simulink model "DFIG_and_BESS_Voltae_Control"  (R2017b)
settings: Solver=ode45  StartTime=0.0  StopTime=6  RelTol=1e-3  EnableMultiTasking=on
undefined symbols (not defined in the file): beta, Cbus, cp_opt_abs, D, D1, D11, Delta, DiscIntNeverNeededParam, f, Fs, fsw, Ion, J, ki_id, ki_idg, ki_iq, ki_iqg, ki_v, kp_id, kp_idg, kp_iq, kp_iqg, kp_v, Kpg, Kqg, lambda_opt, Lg, Lithium, Lm, Lr, Ls, Lsi, N, p, Ps, Radio, Rg, ro, Rr, Rs, sigbuilder_block, sigma, Ts, Vbus_ref, Vdc_bat_ref, Vs
libraries: powerlib x62, powerlib_meascontrol x30, electricdrivelib x1, sps_avr x1
(part 1 of 2)
settings Model: SimulationMode=accelerator  Creator=admin  LastModifiedBy=admin
settings DataIOCC: LimitDataPoints=on  SaveFormat=Array
settings OptimizationCC: EfficientMapNaN2IntZero=off  LifeSpan=inf
settings DebuggingCC: UnderspecifiedInitializationDetection=Classic  MergeDetectMultiDrivingBlocksExec=none  SolverPrmCheckMsg=warning  StateNameClashWarn=warning  SFUnexpectedBacktrackingDiag=warning  SFNoUnconditionalDefaultTransitionDiag=warning  SFExecutionAtInitializationDiag=none
settings HardwareCC: ProdBitPerPointer=32  ProdBitPerSizeT=32  ProdBitPerPtrDiffT=32  ProdLargestAtomicFloat=None  ProdIntDivRoundTo=Undefined  ProdEndianess=Unspecified  ProdWordSize=32  ProdHWDeviceType=32-bit Generic  TargetBitPerPointer=64  TargetBitPerSizeT=64  TargetBitPerPtrDiffT=64  TargetLongLongMode=on  TargetIntDivRoundTo=Zero  TargetEndianess=LittleEndian  TargetWordSize=64  TargetHWDeviceType=MATLAB Host  ProdEqTarget=off
settings ModelReferenceCC: PropagateSignalLabelsOutOfModel=off
settings CodeAppCC: MaxIdLength=128
settings GRTTargetCC: TargetLangStandard=C89/C90 (ANSI)  CombineOutputUpdateFcns=off  GRTInterface=on
settings ConfigComp: CovMetricSettings=dw  CovHtmlReporting=on  CovSaveCumulativeToWorkspaceVar=on  CovSaveSingleToWorkspaceVar=on  CovExternalEMLEnable=off
settings SimscapeCC: SimscapeNormalizeSystem=off

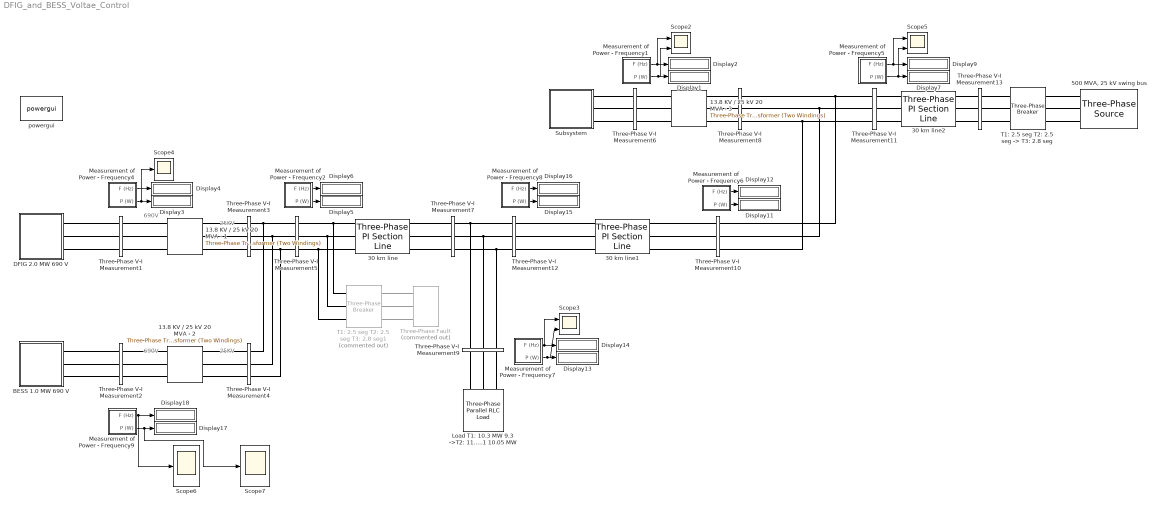
== system DFIG_and_BESS_Voltae_Control ==
  note: 690V
  note: 25KV
  note: 690V
  note: 25KV
  "    T1: 2.5 seg T2: 2.5 seg -> T3: 2.8 seg" : powerlib/Elements/Three-Phase Breaker  InitialState=closed  SwitchA=on  SwitchB=on  SwitchC=on  SwitchTimes=[2.8]  External=off  BreakerResistance=0.01  SnubberResistance=1e6  SnubberCapacitance=inf  Measurements=None
  13.8 KV / 25 kV 20 MVA - 1 : powerlib/Elements/Three-Phase Transformer (Two Windings)  Winding1Connection=Delta (D11)  Winding2Connection=Yg  CoreType=Three single-phase transformers  SetSaturation=off  Hysteresis=off  DataFile='hysteresis'  SetInitialFlux=off  Measurements=None  UNITS=SI  NominalPower=[20e6 f]  Winding1=[25000 0.14881 0.011842]  Winding2=[690 2.624e-05 2.0881e-06]  Rm=89286  Lm=Inf  L0=0.5  Saturation=[0 0;0.47518 112.54;197.99 142.55]  InitialFluxes=[75.026 -75.026 65.648]  MoreParameters=off  BreakLoop=off  DataType=on  TransfoNumber=0
  13.8 KV / 25 kV 20 MVA - 2 : powerlib/Elements/Three-Phase Transformer (Two Windings)  Winding1Connection=Delta (D11)  Winding2Connection=Yg  CoreType=Three single-phase transformers  SetSaturation=off  Hysteresis=off  DataFile='hysteresis'  SetInitialFlux=off  Measurements=None  UNITS=SI  NominalPower="[20e6  f]"  Winding1=[25000 0.14881 0.011842]  Winding2=[690 2.624e-05 2.0881e-06]  Rm=89286  Lm=Inf  L0=0.5  Saturation=[0 0;0.47518 112.54;197.99 142.55]  InitialFluxes=[75.026 -75.026 65.648]  MoreParameters=off  BreakLoop=off  DataType=on  TransfoNumber=0
  13.8 KV / 25 kV 20 MVA - 3 : powerlib/Elements/Three-Phase Transformer (Two Windings)  Winding1Connection=Delta (D11)  Winding2Connection=Yg  CoreType=Three single-phase transformers  SetSaturation=off  Hysteresis=off  DataFile='hysteresis'  SetInitialFlux=off  Measurements=None  UNITS=SI  NominalPower=[20e6 f]  Winding1=[25000 0.14881 0.011842]  Winding2=[13800 2.624e-05 2.0881e-06]  Rm=89286  Lm=Inf  L0=0.5  Saturation=[0 0;0.47518 112.54;197.99 142.55]  InitialFluxes=[75.026 -75.026 65.648]  MoreParameters=off  BreakLoop=off  DataType=on  TransfoNumber=0
  30 km line : powerlib/Elements/Three-Phase PI Section Line  LConnTagsString=a|b|c  RConnTagsString=A|B|C  Frequency=f  Resistances=[0.1153 0.413]  Inductances=[1.05e-3 3.32e-3]  Capacitances=[11.33e-009 5.01e-009]  Length=5
      settings: SourceProductName=Simscape Power Systems
  30 km line1 : powerlib/Elements/Three-Phase PI Section Line  LConnTagsString=a|b|c  RConnTagsString=A|B|C  Frequency=f  Resistances=[0.1153 0.413]  Inductances=[1.05e-3 3.32e-3]  Capacitances=[11.33e-009 5.01e-009]  Length=25
      settings: SourceProductName=Simscape Power Systems
  30 km line2 : powerlib/Elements/Three-Phase PI Section Line  LConnTagsString=a|b|c  RConnTagsString=A|B|C  Frequency=f  Resistances=[0.1153 0.413]  Inductances=[1.05e-3 3.32e-3]  Capacitances=[11.33e-009 5.01e-009]  Length=3
      settings: SourceProductName=Simscape Power Systems
  "500 MVA, 25 kV swing bus" : powerlib/Electrical Sources/Three-Phase Source  InternalConnection=Yg  VoltagePhases=off  Voltage=25e3  PhaseAngle=0  Voltage_phases=[25e3 25e3 25e3]/sqrt(3)  PhaseAngles_phases=[0 -120 +120]  Frequency=f  NonIdealSource=on  SpecifyImpedance=on  Resistance=0  Inductance=47.147e-3  ShortCircuitLevel=500e6  BaseVoltage=25e3  XRratio=100  BusType=swing  Pref=10e3  Qref=0  Prefabc=[10e3, 10e3, 10e3]  Qrefabc=[0, 0, 0]  Qmin=-inf  Qmax=inf
  BESS 1.0 MW 690 V : Subsystem
  DFIG 2.0 MW 690 V : Subsystem
  Display{1..7,9,11..18} (16 alike) : Display
  Load T1: 10.3 MW 9.3 ->T2: 11.1 MW 10 T3: 10.08 MW 9.1 T3.1 10.05 MW : powerlib/Elements/Three-Phase Parallel RLC Load  LConnTagsString=A|B|C  Configuration=Y (grounded)  NominalVoltage=25e3  Vabc=[1e3 1e3 1e3]  Vabcp=[1e3 1e3 1e3]  NominalFrequency=f  UnbalancedPower=off  ActivePower=10.8e6  InductivePower=0  CapacitivePower=0  Pabc=[10e3 9e3 11e3]  QLabc=[100 90 110]  QCabc=[100 90 110]  Pabcp=[10e3 9e3 11e3]  QLabcp=[100 90 110]  QCabcp=[100 90 110]  Measurements=None  LoadType=constant I
  Measurement of Power - Frequency1 : Subsystem
  Measurement of Power - Frequency2 : Subsystem
  Measurement of Power - Frequency4 : Subsystem
  Measurement of Power - Frequency5 : Subsystem
  Measurement of Power - Frequency6 : Subsystem
  Measurement of Power - Frequency7 : Subsystem
  Measurement of Power - Frequency8 : Subsystem
  Measurement of Power - Frequency9 : Subsystem
  Scope2 : Scope  NumInputPorts=2
  Scope3 : Scope  NumInputPorts=2
  Scope4 : Scope
  Scope5 : Scope  NumInputPorts=2
  Scope6 : Scope
  Scope7 : Scope
  Subsystem : Subsystem
  T1: 2.5 seg T2: 2.5 seg T3: 2.8 seg1 : powerlib/Elements/Three-Phase Breaker  Commented=on  InitialState=open  SwitchA=on  SwitchB=on  SwitchC=on  SwitchTimes=[2.8 3 ]  External=off  BreakerResistance=0.01  SnubberResistance=1e6  SnubberCapacitance=inf  Measurements=None
  Three-Phase V-I Measurement1 : powerlib/Measurements/Three-Phase V-I Measurement  VoltageMeasurement=phase-to-ground  SetLabelV=on  LabelV=V_ac_dfig_low  Vpu=off  VpuLL=off  CurrentMeasurement=yes  SetLabelI=on  LabelI=I_ac_dfig_low  Ipu=off  Pbase=100e6  Vbase=500e3  OutputType=Complex  PhasorSimulation=off  PSBequivalent=0
  Three-Phase V-I Measurement10 : powerlib/Measurements/Three-Phase V-I Measurement  VoltageMeasurement=phase-to-ground  SetLabelV=on  LabelV=V_ac_line_4  Vpu=off  VpuLL=off  CurrentMeasurement=yes  SetLabelI=on  LabelI=I_ac_line_4  Ipu=off  Pbase=100e6  Vbase=500e3  OutputType=Complex  PhasorSimulation=off  PSBequivalent=0
  Three-Phase V-I Measurement11 : powerlib/Measurements/Three-Phase V-I Measurement  VoltageMeasurement=phase-to-ground  SetLabelV=on  LabelV=V_ac_syn_slack  Vpu=off  VpuLL=off  CurrentMeasurement=yes  SetLabelI=on  LabelI=I_ac_syn_slack  Ipu=off  Pbase=100e6  Vbase=500e3  OutputType=Complex  PhasorSimulation=off  PSBequivalent=0
  Three-Phase V-I Measurement12 : powerlib/Measurements/Three-Phase V-I Measurement  VoltageMeasurement=phase-to-ground  SetLabelV=on  LabelV=V_ac_line_3  Vpu=off  VpuLL=off  CurrentMeasurement=yes  SetLabelI=on  LabelI=I_ac_line_3  Ipu=off  Pbase=100e6  Vbase=500e3  OutputType=Complex  PhasorSimulation=off  PSBequivalent=0
  Three-Phase V-I Measurement13 : powerlib/Measurements/Three-Phase V-I Measurement  VoltageMeasurement=phase-to-ground  SetLabelV=on  LabelV=V_ac_syn_slack2  Vpu=off  VpuLL=off  CurrentMeasurement=yes  SetLabelI=on  LabelI=I_ac_syn_slack2  Ipu=off  Pbase=100e6  Vbase=500e3  OutputType=Complex  PhasorSimulation=off  PSBequivalent=0
  Three-Phase V-I Measurement2 : powerlib/Measurements/Three-Phase V-I Measurement  VoltageMeasurement=phase-to-ground  SetLabelV=on  LabelV=V_ac_bat_low  Vpu=off  VpuLL=off  CurrentMeasurement=yes  SetLabelI=on  LabelI=I_ac_bat_low  Ipu=off  Pbase=100e6  Vbase=500e3  OutputType=Complex  PhasorSimulation=off  PSBequivalent=0
  Three-Phase V-I Measurement3 : powerlib/Measurements/Three-Phase V-I Measurement  VoltageMeasurement=phase-to-ground  SetLabelV=on  LabelV=V_ac_dfig_H  Vpu=off  VpuLL=off  CurrentMeasurement=yes  SetLabelI=on  LabelI=I_ac_dfig_H  Ipu=off  Pbase=100e6  Vbase=500e3  OutputType=Complex  PhasorSimulation=off  PSBequivalent=0
  Three-Phase V-I Measurement4 : powerlib/Measurements/Three-Phase V-I Measurement  VoltageMeasurement=phase-to-ground  SetLabelV=on  LabelV=V_ac_bat_H  Vpu=off  VpuLL=off  CurrentMeasurement=yes  SetLabelI=on  LabelI=I_ac_bat_H  Ipu=off  Pbase=100e6  Vbase=500e3  OutputType=Complex  PhasorSimulation=off  PSBequivalent=0
  Three-Phase V-I Measurement5 : powerlib/Measurements/Three-Phase V-I Measurement  VoltageMeasurement=phase-to-ground  SetLabelV=on  LabelV=V_ac_line_1  Vpu=off  VpuLL=off  CurrentMeasurement=yes  SetLabelI=on  LabelI=I_ac_line_1  Ipu=off  Pbase=100e6  Vbase=500e3  OutputType=Complex  PhasorSimulation=off  PSBequivalent=0
  Three-Phase V-I Measurement6 : powerlib/Measurements/Three-Phase V-I Measurement  VoltageMeasurement=phase-to-ground  SetLabelV=on  LabelV=V_ac_syn_low  Vpu=off  VpuLL=off  CurrentMeasurement=yes  SetLabelI=on  LabelI=I_ac_syn_low  Ipu=off  Pbase=100e6  Vbase=500e3  OutputType=Complex  PhasorSimulation=off  PSBequivalent=0
  Three-Phase V-I Measurement7 : powerlib/Measurements/Three-Phase V-I Measurement  VoltageMeasurement=phase-to-ground  SetLabelV=on  LabelV=V_ac_line_2  Vpu=off  VpuLL=off  CurrentMeasurement=yes  SetLabelI=on  LabelI=I_ac_line_2  Ipu=off  Pbase=100e6  Vbase=500e3  OutputType=Complex  PhasorSimulation=off  PSBequivalent=0
  Three-Phase V-I Measurement8 : powerlib/Measurements/Three-Phase V-I Measurement  VoltageMeasurement=phase-to-ground  SetLabelV=on  LabelV=V_ac_syn_H  Vpu=off  VpuLL=off  CurrentMeasurement=yes  SetLabelI=on  LabelI=I_ac_syn_H  Ipu=off  Pbase=100e6  Vbase=500e3  OutputType=Complex  PhasorSimulation=off  PSBequivalent=0
  Three-Phase V-I Measurement9 : powerlib/Measurements/Three-Phase V-I Measurement  VoltageMeasurement=phase-to-ground  SetLabelV=on  LabelV=V_ac_load  Vpu=off  VpuLL=off  CurrentMeasurement=yes  SetLabelI=on  LabelI=I_ac_load  Ipu=off  Pbase=100e6  Vbase=500e3  OutputType=Complex  PhasorSimulation=off  PSBequivalent=0
  Three-Phase Fault : powerlib/Elements/Three-Phase Fault  Commented=on  InitialStates=1  FaultA=on  FaultB=on  FaultC=on  GroundFault=on  SwitchTimes="[1/60  5/60]"  External=off  SwitchStatus=NaN  FaultResistance=0.001  GroundResistance=0.01  SnubberResistance=1e6  SnubberCapacitance=inf  Measurements=None
  powergui : powerlib/powergui  Priority=1  SimulationMode=Discrete  SampleTime=Ts  frequency=60  Iterations=50  frequencyindice=0  Pbase=100e6  ErrMax=1e-4  UnitsV=kV  UnitsW=MW  buscounter=0  FunctionMessages=off  echomessages=off  EnableUseOfTLC=off  CurrentSourceSwitches=off  DisableSnubberDevices=off  DisableRonSwitches=off  DisableVfSwitches=off  DisplayEquations=off  SolverType=Tustin  Interpol=off  ExternalGateDelay=off  methode=off  Ts=0  x0status=blocks  SPID=off  SwTol=0  HookPort=off  RestoreLinks=warning  ResistiveCurrentMeasurement=off  Frange=[0:2:500]  Ylog=off  Xlog=on  ShowGrid=off  save=off  variable=ZData  structure=0  ZoomFFT=off  StartTime=0.0  cycles=1  DisplayStyle=1  fundamental=60  FreqAxis=off  MaxFrequency=1000  frequencyindicesteady=1  RmsSteady=1  display=off
  wires:
  Measurement of Power - Frequency1/1(F (Hz)) -> Scope2/1, Display2/1
  Measurement of Power - Frequency1/2(P (W)) -> Display1/1, Scope2/2
  Measurement of Power - Frequency4/2(P (W)) -> Scope4/1, Display3/1
  Measurement of Power - Frequency4/1(F (Hz)) -> Display4/1
  Measurement of Power - Frequency2/2(P (W)) -> Display5/1
  Measurement of Power - Frequency2/1(F (Hz)) -> Display6/1
  Measurement of Power - Frequency5/2(P (W)) -> Display7/1, Scope5/2
  Measurement of Power - Frequency5/1(F (Hz)) -> Display9/1, Scope5/1
  Measurement of Power - Frequency6/1(F (Hz)) -> Display12/1
  Measurement of Power - Frequency6/2(P (W)) -> Display11/1
  Measurement of Power - Frequency7/2(P (W)) -> Scope3/2, Display13/1
  Measurement of Power - Frequency7/1(F (Hz)) -> Display14/1, Scope3/1
  Measurement of Power - Frequency8/2(P (W)) -> Display15/1
  Measurement of Power - Frequency8/1(F (Hz)) -> Display16/1
  Measurement of Power - Frequency9/1(F (Hz)) -> Display18/1, Scope6/1
  Measurement of Power - Frequency9/2(P (W)) -> Scope7/1, Display17/1
  connections:
  BESS 1.0 MW 690 V/RConn1 -- Three-Phase V-I Measurement2/LConn1
  BESS 1.0 MW 690 V/RConn2 -- Three-Phase V-I Measurement2/LConn2
  BESS 1.0 MW 690 V/RConn3 -- Three-Phase V-I Measurement2/LConn3
  DFIG 2.0 MW 690 V/RConn3 -- Three-Phase V-I Measurement1/LConn3
  DFIG 2.0 MW 690 V/RConn1 -- Three-Phase V-I Measurement1/LConn1
  DFIG 2.0 MW 690 V/RConn2 -- Three-Phase V-I Measurement1/LConn2
  Three-Phase V-I Measurement1/RConn1 -- 13.8 KV / 25 kV 20 MVA - 1/RConn1
  Three-Phase V-I Measurement1/RConn2 -- 13.8 KV / 25 kV 20 MVA - 1/RConn2
  Three-Phase V-I Measurement1/RConn3 -- 13.8 KV / 25 kV 20 MVA - 1/RConn3
  13.8 KV / 25 kV 20 MVA - 1/LConn1 -- Three-Phase V-I Measurement3/LConn1
  13.8 KV / 25 kV 20 MVA - 1/LConn2 -- Three-Phase V-I Measurement3/LConn2
  13.8 KV / 25 kV 20 MVA - 1/LConn3 -- Three-Phase V-I Measurement3/LConn3
  13.8 KV / 25 kV 20 MVA - 2/LConn1 -- Three-Phase V-I Measurement4/LConn1
  13.8 KV / 25 kV 20 MVA - 2/LConn2 -- Three-Phase V-I Measurement4/LConn2
  13.8 KV / 25 kV 20 MVA - 2/LConn3 -- Three-Phase V-I Measurement4/LConn3
  Three-Phase V-I Measurement2/RConn1 -- 13.8 KV / 25 kV 20 MVA - 2/RConn1
  Three-Phase V-I Measurement2/RConn2 -- 13.8 KV / 25 kV 20 MVA - 2/RConn2
  Three-Phase V-I Measurement2/RConn3 -- 13.8 KV / 25 kV 20 MVA - 2/RConn3
  Three-Phase V-I Measurement5/LConn1 -- Three-Phase V-I Measurement4/RConn1 -- Three-Phase V-I Measurement3/RConn1
  Three-Phase V-I Measurement5/LConn2 -- Three-Phase V-I Measurement4/RConn2 -- Three-Phase V-I Measurement3/RConn2
  Three-Phase V-I Measurement5/LConn3 -- Three-Phase V-I Measurement4/RConn3 -- Three-Phase V-I Measurement3/RConn3
  30 km line/LConn1 -- T1: 2.5 seg T2: 2.5 seg T3: 2.8 seg1/LConn1 -- Three-Phase V-I Measurement5/RConn1
  30 km line/LConn2 -- T1: 2.5 seg T2: 2.5 seg T3: 2.8 seg1/LConn2 -- Three-Phase V-I Measurement5/RConn2
  30 km line/LConn3 -- T1: 2.5 seg T2: 2.5 seg T3: 2.8 seg1/LConn3 -- Three-Phase V-I Measurement5/RConn3
  Three-Phase V-I Measurement8/LConn1 -- 13.8 KV / 25 kV 20 MVA - 3/LConn1
  Three-Phase V-I Measurement8/LConn2 -- 13.8 KV / 25 kV 20 MVA - 3/LConn2
  Three-Phase V-I Measurement8/LConn3 -- 13.8 KV / 25 kV 20 MVA - 3/LConn3
  Three-Phase V-I Measurement6/RConn1 -- 13.8 KV / 25 kV 20 MVA - 3/RConn1
  Three-Phase V-I Measurement6/RConn2 -- 13.8 KV / 25 kV 20 MVA - 3/RConn2
  Three-Phase V-I Measurement6/RConn3 -- 13.8 KV / 25 kV 20 MVA - 3/RConn3
  30 km line1/RConn2 -- Three-Phase V-I Measurement10/LConn2
  30 km line1/RConn1 -- Three-Phase V-I Measurement10/LConn1
  30 km line1/RConn3 -- Three-Phase V-I Measurement10/LConn3
  Three-Phase V-I Measurement10/RConn3 -- Three-Phase V-I Measurement8/RConn3 -- Three-Phase V-I Measurement11/LConn3
  Three-Phase V-I Measurement10/RConn2 -- Three-Phase V-I Measurement8/RConn2 -- Three-Phase V-I Measurement11/LConn2
  Three-Phase V-I Measurement10/RConn1 -- Three-Phase V-I Measurement8/RConn1 -- Three-Phase V-I Measurement11/LConn1
  Load T1: 10.3 MW 9.3 ->T2: 11.1 MW 10 T3: 10.08 MW 9.1 T3.1 10.05 MW/LConn1 -- Three-Phase V-I Measurement9/RConn3
  Load T1: 10.3 MW 9.3 ->T2: 11.1 MW 10 T3: 10.08 MW 9.1 T3.1 10.05 MW/LConn2 -- Three-Phase V-I Measurement9/RConn2
  Load T1: 10.3 MW 9.3 ->T2: 11.1 MW 10 T3: 10.08 MW 9.1 T3.1 10.05 MW/LConn3 -- Three-Phase V-I Measurement9/RConn1
  30 km line/RConn1 -- Three-Phase V-I Measurement7/LConn1
  30 km line/RConn2 -- Three-Phase V-I Measurement7/LConn2
  30 km line/RConn3 -- Three-Phase V-I Measurement7/LConn3
  Three-Phase V-I Measurement7/RConn1 -- Three-Phase V-I Measurement9/LConn3 -- Three-Phase V-I Measurement12/LConn1
  Three-Phase V-I Measurement7/RConn2 -- Three-Phase V-I Measurement9/LConn2 -- Three-Phase V-I Measurement12/LConn2
  Three-Phase V-I Measurement7/RConn3 -- Three-Phase V-I Measurement9/LConn1 -- Three-Phase V-I Measurement12/LConn3
  Three-Phase V-I Measurement12/RConn1 -- 30 km line1/LConn1
  Three-Phase V-I Measurement12/RConn2 -- 30 km line1/LConn2
  Three-Phase V-I Measurement12/RConn3 -- 30 km line1/LConn3
  Subsystem/LConn1 -- Three-Phase V-I Measurement6/LConn1
  Subsystem/LConn2 -- Three-Phase V-I Measurement6/LConn2
  Subsystem/LConn3 -- Three-Phase V-I Measurement6/LConn3
  "    T1: 2.5 seg T2: 2.5 seg -> T3: 2.8 seg"/RConn1 -- "500 MVA, 25 kV swing bus"/RConn1
  "    T1: 2.5 seg T2: 2.5 seg -> T3: 2.8 seg"/RConn2 -- "500 MVA, 25 kV swing bus"/RConn2
  "    T1: 2.5 seg T2: 2.5 seg -> T3: 2.8 seg"/RConn3 -- "500 MVA, 25 kV swing bus"/RConn3
  30 km line2/RConn1 -- Three-Phase V-I Measurement13/LConn1
  Three-Phase V-I Measurement13/RConn2 -- "    T1: 2.5 seg T2: 2.5 seg -> T3: 2.8 seg"/LConn2
  Three-Phase V-I Measurement13/RConn3 -- "    T1: 2.5 seg T2: 2.5 seg -> T3: 2.8 seg"/LConn3
  Three-Phase V-I Measurement13/RConn1 -- "    T1: 2.5 seg T2: 2.5 seg -> T3: 2.8 seg"/LConn1
  30 km line2/RConn3 -- Three-Phase V-I Measurement13/LConn3
  30 km line2/RConn2 -- Three-Phase V-I Measurement13/LConn2
  30 km line2/LConn1 -- Three-Phase V-I Measurement11/RConn1
  30 km line2/LConn2 -- Three-Phase V-I Measurement11/RConn2
  30 km line2/LConn3 -- Three-Phase V-I Measurement11/RConn3
  Three-Phase Fault/LConn1 -- T1: 2.5 seg T2: 2.5 seg T3: 2.8 seg1/RConn1
  Three-Phase Fault/LConn2 -- T1: 2.5 seg T2: 2.5 seg T3: 2.8 seg1/RConn2
  Three-Phase Fault/LConn3 -- T1: 2.5 seg T2: 2.5 seg T3: 2.8 seg1/RConn3

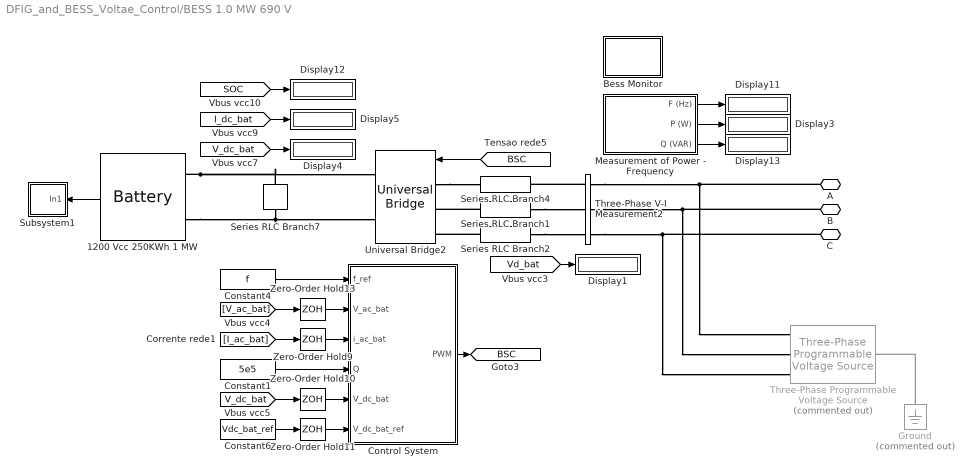
== system DFIG_and_BESS_Voltae_Control/BESS 1.0 MW 690 V ==
  "1200 Vcc 250KWh 1 MW " : electricdrivelib/Extra Sources/Battery  BatType=Lithium-Ion  ShowTempParam=off  ThermalPreset=no  ShowAgeParam=off  NomV=1200  NomQ=100  SOC=71.5  Batt_Tr=30  PresetModel=on  MaxQ=100  MinV=900  FullV=1396.7846  Dis_rate=43.4783  R=0.12  Normal_OP=90.4348  expZone="[1296.463      4.9130435]"  current=[6.5 13 32.5]  Units=Time  Tci=20  NomT=25  T2=0  MaxQ2=2.208  FullV2=3.45  Normal_OP2=2.8  expZone2="[3.22        0.23]"  Rca=0.6  ti=1000  Dp=0  Neq0=0  Tsim=1e6  Ta1=25  Qeol=5.4*0.9  Reol=0.013333*1.2  Char_age=[2.3478, 3]  Dis_age=[2.3478, 10]  N1=1500  N2=10500  N3=1000  N4=1400  Ta2=45  N5=950
  Bess Monitor : Subsystem
  Constant1 : Constant  Value=5e5
  Constant4 : Constant  Value=f
  Constant6 : Constant  Value=Vdc_bat_ref
  Control System : Subsystem
  Display{1,3..5,11..13} (7 alike) : Display
  Ground : powerlib/Elements/Ground  Commented=on  LConnTagsString=a
  Measurement of Power - Frequency : Subsystem
  Series RLC Branch1 : powerlib/Elements/Series RLC Branch  LConnTagsString=__new0  RConnTagsString=__new0  BranchType=RL  Resistance=20e-5  Inductance=600e-6  SetiL0=off  InitialCurrent=0  Capacitance=0  Setx0=off  InitialVoltage=0  Measurements=None
  Series RLC Branch2 : powerlib/Elements/Series RLC Branch  LConnTagsString=__new0  RConnTagsString=__new0  BranchType=RL  Resistance=20e-5  Inductance=600e-6  SetiL0=off  InitialCurrent=0  Capacitance=0  Setx0=off  InitialVoltage=0  Measurements=None
  Series RLC Branch4 : powerlib/Elements/Series RLC Branch  LConnTagsString=__new0  RConnTagsString=__new0  BranchType=RL  Resistance=20e-5  Inductance=600e-6  SetiL0=off  InitialCurrent=0  Capacitance=0  Setx0=off  InitialVoltage=0  Measurements=None
  Series RLC Branch7 : powerlib/Elements/Series RLC Branch  LConnTagsString=__new0  RConnTagsString=__new0  BranchType=C  Resistance=1  Inductance=1e-3  SetiL0=off  InitialCurrent=0  Capacitance=15e-3  Setx0=off  InitialVoltage=0  Measurements=Branch voltage
  Subsystem1 : Subsystem
  Three-Phase Programmable Voltage Source : powerlib/Electrical Sources/Three-Phase Programmable Voltage Source  Commented=on  PositiveSequence="[Vs  0 f]"  VariationEntity=None  VariationType=Table of time-amplitude pairs  VariationTypeAlt=Step  VariationStep=-0.8  VariationRate=10  VariationMagnitude=0.3  VariationFrequency=2  VariationTiming=[0.2 3]  VariationPhaseA=off  Amplitudes=[1 0.8 1.2 1.0]  TimeValues=[0 0.1 0.15 0.2]  HarmonicGeneration=off  HarmonicA=[3 0.2 -25 0]  HarmonicB=[2 0.15 35 2]  Timing="[0.05  3]"  BusType=swing  Pref=0  Qref=0  Qmin=-inf  Qmax=inf
  Three-Phase V-I Measurement2 : powerlib/Measurements/Three-Phase V-I Measurement  VoltageMeasurement=phase-to-ground  SetLabelV=on  LabelV=V_ac_bat  Vpu=off  VpuLL=off  CurrentMeasurement=yes  SetLabelI=on  LabelI=I_ac_bat  Ipu=off  Pbase=100e6  Vbase=500e3  OutputType=Complex  PhasorSimulation=off  PSBequivalent=0
  Universal Bridge2 : powerlib/Power Electronics/Universal Bridge  Arms=3  SnubberResistance=1e5  SnubberCapacitance=inf  Device=Ideal Switches  Ron=1e-3  Lon=0  ForwardVoltages="[  0  0  ]"  ForwardVoltage=0  GTOparameters=[ 10e-6 , 20e-6 ]  IGBTparameters=[ 1e-6 , 2e-6 ]  Measurements=None  Measurements_2=None  converterType=Rectifier
  Zero-Order Hold{9..11,13} (4 alike) : ZeroOrderHold  SampleTime=1/fsw
  A : PMIOPort  Port=1  Side=Right
  B : PMIOPort  Port=2  Side=Right
  C : PMIOPort  Port=3  Side=Right
  tag scope: BSC=global
  wires:
  Zero-Order Hold10/1 -> Control System/5(V_dc_bat)
  Constant4/1 -> Control System/1(f_ref)
  [V_dc_bat] -> Zero-Order Hold10/1
  [I_dc_bat] -> Display5/1
  Control System/1(PWM) -> [BSC]
  Zero-Order Hold11/1 -> Control System/6(V_dc_bat_ref)
  [V_dc_bat] -> Display4/1
  "1200 Vcc 250KWh 1 MW "/1 -> Subsystem1/1(In1)
  Zero-Order Hold13/1 -> Control System/2("V_ac_bat ")
  [V_ac_bat] -> Zero-Order Hold13/1
  Constant6/1 -> Zero-Order Hold11/1
  Zero-Order Hold9/1 -> Control System/3(i_ac_bat)
  [BSC] -> Universal Bridge2/1
  Constant1/1 -> Control System/4(Q)
  [I_ac_bat] -> Zero-Order Hold9/1
  Measurement of Power - Frequency/2(P (W)) -> Display3/1
  Measurement of Power - Frequency/1(F (Hz)) -> Display11/1
  Measurement of Power - Frequency/3(Q (VAR)) -> Display13/1
  [SOC] -> Display12/1
  [Vd_bat] -> Display1/1
  connections:
  Series RLC Branch7/RConn1 -- "1200 Vcc 250KWh 1 MW "/LConn2 -- Universal Bridge2/RConn2
  "1200 Vcc 250KWh 1 MW "/LConn1 -- Series RLC Branch7/LConn1 -- Universal Bridge2/RConn1
  Universal Bridge2/LConn1 -- Series RLC Branch4/LConn1
  Three-Phase V-I Measurement2/LConn1 -- Series RLC Branch4/RConn1
  Series RLC Branch2/LConn1 -- Universal Bridge2/LConn3
  Series RLC Branch1/RConn1 -- Three-Phase V-I Measurement2/LConn2
  Series RLC Branch1/LConn1 -- Universal Bridge2/LConn2
  Series RLC Branch2/RConn1 -- Three-Phase V-I Measurement2/LConn3
  Three-Phase V-I Measurement2/RConn1 -- Three-Phase Programmable Voltage Source/RConn1 -- A/RConn1
  Three-Phase V-I Measurement2/RConn2 -- Three-Phase Programmable Voltage Source/RConn2 -- B/RConn1
  Three-Phase V-I Measurement2/RConn3 -- Three-Phase Programmable Voltage Source/RConn3 -- C/RConn1
  Ground/LConn1 -- Three-Phase Programmable Voltage Source/LConn1

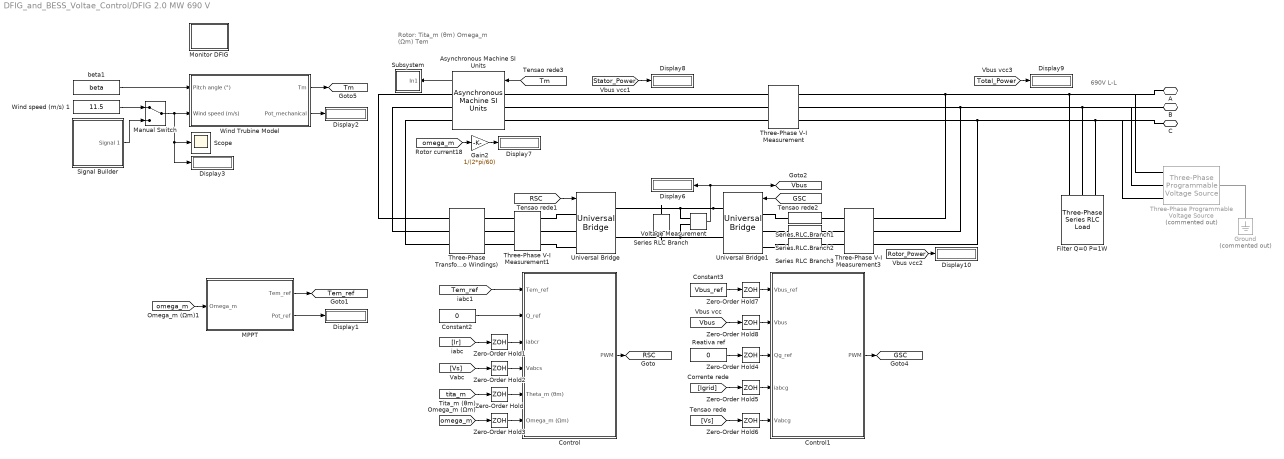
== system DFIG_and_BESS_Voltae_Control/DFIG 2.0 MW 690 V ==
  note: 690V L-L
  note: Rotor:
      | Tita_m (θm)
      | Omega_m (Ωm)
      | Tem
  Asynchronous Machine SI Units : powerlib/Machines/Asynchronous Machine SI Units  RotorType=Wound  PresetModel=No  MechanicalLoad=Torque Tm  ShowDetailedParameters=on  ReferenceFrame=Rotor  Units=SI  MeasurementBus=off  NominalParameters=[ Ps Vs f ]  Stator=[ Rs , Lsi]  Rotor=[ Rr , Lsi]  Cage1=[ 0.022 0.226/377]  Cage2=[ 0.022 0.226/377]  Lm=Lm  Mechanical=[ J D 2 ]  PolePairs=2  InitialConditions=[1 0 0 0 0 0 0 0]  SimulateSaturation=off  Saturation=[14.03593122, 27.81365428, 53.79336849, 72.68890987, 97.98006896, 148.6815601, 215.7428561, 302.9841135, 420.4778367 ; 230, 322, 414, 460, 506, 552, 598, 644, 690]  LoadFlowParameters=1492000  TsPowergui=0  TsBlock=-1  IterativeModel=Trapezoidal non iterative  IterativeDiscreteModel=Trapezoidal non iterative  Pmec=0
  Constant2 : Constant  Value=0
  Constant3 : Constant  Value=Vbus_ref
  Control : Subsystem
  Control1 : Subsystem
  Display{1..3,6..10} (8 alike) : Display
  Filter Q=0 P=1W : powerlib/Elements/Three-Phase Series RLC Load  LConnTagsString=A|B|C  Configuration=Y (grounded)  NominalVoltage=Vs  Vabc=[1e3 1e3 1e3]  Vabcp=[1e3 1e3 1e3]  NominalFrequency=f  UnbalancedPower=off  ActivePower=1  InductivePower=0  CapacitivePower=0  Pabc=[10e3 9e3 11e3]  QLabc=[100 90 110]  QCabc=[100 90 110]  Pabcp=[10e3 9e3 11e3]  QLabcp=[100 90 110]  QCabcp=[100 90 110]  Measurements=None  LoadType=constant Z
  Gain2 : Gain  Gain=1/(2*pi/60)
  Ground : powerlib/Elements/Ground  Commented=on  LConnTagsString=a
  MPPT : Subsystem
  Manual Switch : ManualSwitch
  Monitor DFIG : Subsystem
  Reativa ref : Constant  Value=0
  Scope : Scope
  Series RLC Branch : powerlib/Elements/Series RLC Branch  LConnTagsString=__new0  RConnTagsString=__new0  BranchType=C  Resistance=1  Inductance=1e-3  SetiL0=off  InitialCurrent=0  Capacitance=Cbus  Setx0=off  InitialVoltage=0  Measurements=Branch voltage
  Series RLC Branch1 : powerlib/Elements/Series RLC Branch  LConnTagsString=__new0  RConnTagsString=__new0  BranchType=RL  Resistance=Rg  Inductance=Lg  SetiL0=off  InitialCurrent=0  Capacitance=0  Setx0=off  InitialVoltage=0  Measurements=None
  Series RLC Branch2 : powerlib/Elements/Series RLC Branch  LConnTagsString=__new0  RConnTagsString=__new0  BranchType=RL  Resistance=Rg  Inductance=Lg  SetiL0=off  InitialCurrent=0  Capacitance=0  Setx0=off  InitialVoltage=0  Measurements=None
  Series RLC Branch3 : powerlib/Elements/Series RLC Branch  LConnTagsString=__new0  RConnTagsString=__new0  BranchType=RL  Resistance=Rg  Inductance=Lg  SetiL0=off  InitialCurrent=0  Capacitance=0  Setx0=off  InitialVoltage=0  Measurements=None
  Signal Builder : Subsystem  Tag=STV Subsys  LoadFcn=sigbuilder_block('load');  StartFcn=sigbuilder_block('start');  StopFcn=sigbuilder_block('stop');  ClipboardFcn=sigbuilder_block('clipboard');  mask(Sigbuilder block){tuvar=[0:10]}
      mask help: Simulink:masks:SigbuilderBlock_MD
      mask init:
      | if ~strcmp(get_param(bdroot(gcbh),'SimulationStatus'),'stopped') tuvar = sigbuilder_block('maskInit'); end
      settings: CopyFcn=sigbuilder_block('copy');  DeleteFcn=sigbuilder_block('delete');  ModelCloseFcn=sigbuilder_block('modelClose');  PreSaveFcn=sigbuilder_block('preSave');  PauseFcn=sigbuilder_block('pause');  ContinueFcn=sigbuilder_block('continue');  NameChangeFcn=sigbuilder_block('namechange');  OpenFcn=sigbuilder_block('open',[6 22.5 1012.5 455.25 ]);  CloseFcn=sigbuilder_block('close');
      mask Display: plot(0, 0, 100, 100,[2, 2, 32, 32, 2], [68, 8, 8, 68, 68],[32, 2], [38, 38], [32, 19, 2],[53, 60, 44], [32, 17, 17, 2],[16, 16, 31, 31]);txt = getActiveGroup(gcbh);text(2, 100, txt,'verticalAlignment', 'top');
  Subsystem : Subsystem
  Three-Phase Programmable Voltage Source : powerlib/Electrical Sources/Three-Phase Programmable Voltage Source  Commented=on  PositiveSequence="[Vs  0 f]"  VariationEntity=Frequency  VariationType=Table of time-amplitude pairs  VariationTypeAlt=Step  VariationStep=-0.8  VariationRate=10  VariationMagnitude=0.3  VariationFrequency=2  VariationTiming=[0.2 3]  VariationPhaseA=off  Amplitudes=[1 0.8 1.2 1.0]  TimeValues=[0 0.1 0.15 0.2]  HarmonicGeneration=off  HarmonicA=[3 0.2 -25 0]  HarmonicB=[2 0.15 35 2]  Timing="[0.05  3]"  BusType=swing  Pref=0  Qref=0  Qmin=-inf  Qmax=inf
  Three-Phase Transformer (Two Windings) : powerlib/Elements/Three-Phase Transformer (Two Windings)  Winding1Connection=Y  Winding2Connection=Y  CoreType=Three single-phase transformers  SetSaturation=off  Hysteresis=off  DataFile='hysteresis'  SetInitialFlux=off  Measurements=None  UNITS=SI  NominalPower=[ Ps , f]  Winding1=[Vs 0 0]  Winding2=[Vs/u 0 0]  Rm=1.0805e+06  Lm=2866  L0=0.5  Saturation=[0 0;0.66653 1910.3;277.72 2419.7]  InitialFluxes=[1273.5 -1273.5 1114.3]  MoreParameters=off  BreakLoop=off  DataType=on  TransfoNumber=1
  Three-Phase V-I Measurement : powerlib/Measurements/Three-Phase V-I Measurement  VoltageMeasurement=phase-to-ground  SetLabelV=on  LabelV=Vs  Vpu=off  VpuLL=off  CurrentMeasurement=yes  SetLabelI=on  LabelI=Is  Ipu=off  Pbase=100e6  Vbase=500e3  OutputType=Complex  PhasorSimulation=off  PSBequivalent=0
  Three-Phase V-I Measurement1 : powerlib/Measurements/Three-Phase V-I Measurement  VoltageMeasurement=phase-to-phase  SetLabelV=on  LabelV=Vr  Vpu=off  VpuLL=off  CurrentMeasurement=yes  SetLabelI=on  LabelI=Ir  Ipu=off  Pbase=100e6  Vbase=500e3  OutputType=Complex  PhasorSimulation=off  PSBequivalent=0
  Three-Phase V-I Measurement3 : powerlib/Measurements/Three-Phase V-I Measurement  VoltageMeasurement=phase-to-ground  SetLabelV=on  LabelV=Vgrid  Vpu=off  VpuLL=off  CurrentMeasurement=yes  SetLabelI=on  LabelI=Igrid  Ipu=off  Pbase=100e6  Vbase=500e3  OutputType=Complex  PhasorSimulation=off  PSBequivalent=0
  Universal Bridge : powerlib/Power Electronics/Universal Bridge  Arms=3  SnubberResistance=1e5  SnubberCapacitance=inf  Device=Ideal Switches  Ron=1e-3  Lon=0  ForwardVoltages="[  0  0  ]"  ForwardVoltage=0  GTOparameters=[ 10e-6 , 20e-6 ]  IGBTparameters=[ 1e-6 , 2e-6 ]  Measurements=None  Measurements_2=None  converterType=Rectifier
  Universal Bridge1 : powerlib/Power Electronics/Universal Bridge  Arms=3  SnubberResistance=1e5  SnubberCapacitance=inf  Device=Ideal Switches  Ron=1e-3  Lon=0  ForwardVoltages="[  0  0  ]"  ForwardVoltage=0  GTOparameters=[ 10e-6 , 20e-6 ]  IGBTparameters=[ 1e-6 , 2e-6 ]  Measurements=None  Measurements_2=None  converterType=Rectifier
  Voltage Measurement : powerlib/Measurements/Voltage Measurement  PhasorSimulation=off  OutputType=Complex  PSBequivalent=0
  Wind Trubine Model : Subsystem
  Wind speed (m/s) 1 : Constant  Value=11.5
  Zero-Order Hold{,1..8} (9 alike) : ZeroOrderHold  SampleTime=1/fsw
  beta1 : Constant  Value=beta
  A : PMIOPort  Port=1  Side=Right
  B : PMIOPort  Port=2  Side=Right
  C : PMIOPort  Port=3  Side=Right
  tag scope: GSC=global, RSC=global, Tem_ref=global, Tm=global, Vbus=global
  wires:
  [Igrid] -> Zero-Order Hold5/1
  beta1/1 -> Wind Trubine Model/1(Pitch angle (°))
  Constant3/1 -> Zero-Order Hold7/1
  MPPT/1(Tem_ref) -> [Tem_ref]
  Wind Trubine Model/1(Tm) -> [Tm]
  [Stator_Power] -> Display8/1
  [Tm] -> Asynchronous Machine SI Units/1
  MPPT/2("Pot_ref ") -> Display1/1
  Reativa ref/1 -> Zero-Order Hold4/1
  [GSC] -> Universal Bridge1/1
  Wind Trubine Model/2(Pot_mechanical) -> Display2/1
  [omega_m] -> MPPT/1(Omega_m)
  Control/1(PWM) -> [RSC]
  [tita_m] -> Zero-Order Hold/1
  [Tem_ref] -> Control/1(Tem_ref)
  [Rotor_Power] -> Display10/1
  [omega_m] -> Gain2/1
  [Vs] -> Zero-Order Hold2/1
  Asynchronous Machine SI Units/1 -> Subsystem/1(In1)
  Zero-Order Hold/1 -> Control/5(Theta_m (θm))
  Zero-Order Hold2/1 -> Control/4(Vabcs)
  [omega_m] -> Zero-Order Hold3/1
  Gain2/1 -> Display7/1
  Zero-Order Hold1/1 -> Control/3(iabcr)
  Constant2/1 -> Control/2(Q_ref)
  [Vbus] -> Zero-Order Hold8/1
  Zero-Order Hold7/1 -> Control1/1(Vbus_ref)
  [RSC] -> Universal Bridge/1
  Zero-Order Hold3/1 -> Control/6("Omega_m (Ωm) ")
  [Ir] -> Zero-Order Hold1/1
  [Vs] -> Zero-Order Hold6/1
  [Total_Power] -> Display9/1
  Zero-Order Hold6/1 -> Control1/5("Vabcg ")
  Zero-Order Hold5/1 -> Control1/4(iabcg)
  Voltage Measurement/1 -> Display6/1, [Vbus]
  Zero-Order Hold4/1 -> Control1/3(Qg_ref)
  Control1/1(PWM) -> [GSC]
  Zero-Order Hold8/1 -> Control1/2(Vbus)
  Manual Switch/1 -> Display3/1, Scope/1, Wind Trubine Model/2(Wind speed (m/s))
  Wind speed (m/s) 1/1 -> Manual Switch/1
  Signal Builder/1(Signal 1) -> Manual Switch/2
  connections:
  Three-Phase V-I Measurement/RConn2 -- Three-Phase Programmable Voltage Source/RConn2 -- B/RConn1 -- Filter Q=0 P=1W/LConn2 -- Three-Phase V-I Measurement3/RConn2
  Three-Phase V-I Measurement/RConn1 -- Three-Phase Programmable Voltage Source/RConn1 -- A/RConn1 -- Filter Q=0 P=1W/LConn1 -- Three-Phase V-I Measurement3/RConn1
  Voltage Measurement/LConn2 -- Universal Bridge1/RConn2 -- Universal Bridge/RConn2 -- Series RLC Branch/RConn1
  Universal Bridge1/RConn1 -- Voltage Measurement/LConn1 -- Universal Bridge/RConn1 -- Series RLC Branch/LConn1
  Three-Phase V-I Measurement/RConn3 -- Three-Phase Programmable Voltage Source/RConn3 -- C/RConn1 -- Filter Q=0 P=1W/LConn3 -- Three-Phase V-I Measurement3/RConn3
  Three-Phase Transformer (Two Windings)/LConn2 -- Asynchronous Machine SI Units/RConn2
  Three-Phase Transformer (Two Windings)/LConn3 -- Asynchronous Machine SI Units/RConn3
  Three-Phase V-I Measurement3/LConn2 -- Series RLC Branch2/RConn1
  Three-Phase V-I Measurement1/LConn1 -- Universal Bridge/LConn1
  Three-Phase V-I Measurement/LConn1 -- Asynchronous Machine SI Units/LConn1
  Three-Phase V-I Measurement3/LConn3 -- Series RLC Branch3/RConn1
  Three-Phase Transformer (Two Windings)/LConn1 -- Asynchronous Machine SI Units/RConn1
  Three-Phase V-I Measurement/LConn3 -- Asynchronous Machine SI Units/LConn3
  Three-Phase V-I Measurement3/LConn1 -- Series RLC Branch1/RConn1
  Three-Phase Transformer (Two Windings)/RConn3 -- Three-Phase V-I Measurement1/RConn3
  Three-Phase V-I Measurement1/LConn3 -- Universal Bridge/LConn3
  Universal Bridge1/LConn1 -- Series RLC Branch1/LConn1
  Three-Phase V-I Measurement1/LConn2 -- Universal Bridge/LConn2
  Three-Phase Transformer (Two Windings)/RConn2 -- Three-Phase V-I Measurement1/RConn2
  Universal Bridge1/LConn3 -- Series RLC Branch3/LConn1
  Three-Phase V-I Measurement/LConn2 -- Asynchronous Machine SI Units/LConn2
  Universal Bridge1/LConn2 -- Series RLC Branch2/LConn1
  Three-Phase Transformer (Two Windings)/RConn1 -- Three-Phase V-I Measurement1/RConn1
  Ground/LConn1 -- Three-Phase Programmable Voltage Source/LConn1

== system DFIG_and_BESS_Voltae_Control/Measurement of Power - Frequency1 ==
  PLL (3ph)1 : powerlib_meascontrol/PLL/PLL (3ph)  Commented=on  Fmin=45  Par_Init=[0, f]  ParK=[180, 3200, 1]  TcD=1e-4  MaxRateChangeFreq=12  FilterCutOffFreq=25  Ts=0  AGC=on
  "Power (3ph, Instantaneous)1" : powerlib_meascontrol/Measurements/Power (3ph, Instantaneous)
      settings: SourceProductName=Simscape Power Systems
  F (Hz) : Outport
  P (W) : Outport  Port=2
  wires:
  [I_ac_syn_low] -> "Power (3ph, Instantaneous)1"/2
  PLL (3ph)1/1 -> F (Hz)/1
  "Power (3ph, Instantaneous)1"/1 -> P (W)/1  "Pot"
  [V_ac_syn_low] -> PLL (3ph)1/1, "Power (3ph, Instantaneous)1"/1

== system DFIG_and_BESS_Voltae_Control/Measurement of Power - Frequency2 ==
  PLL (3ph)1 : powerlib_meascontrol/PLL/PLL (3ph)  Commented=on  Fmin=45  Par_Init=[0, f]  ParK=[180, 3200, 1]  TcD=1e-4  MaxRateChangeFreq=12  FilterCutOffFreq=25  Ts=0  AGC=on
  "Power (3ph, Instantaneous)1" : powerlib_meascontrol/Measurements/Power (3ph, Instantaneous)
      settings: SourceProductName=Simscape Power Systems
  F (Hz) : Outport
  P (W) : Outport  Port=2
  wires:
  [I_ac_line_1] -> "Power (3ph, Instantaneous)1"/2
  PLL (3ph)1/1 -> F (Hz)/1
  "Power (3ph, Instantaneous)1"/1 -> P (W)/1  "Pot"
  [V_ac_line_1] -> PLL (3ph)1/1, "Power (3ph, Instantaneous)1"/1

== system DFIG_and_BESS_Voltae_Control/Measurement of Power - Frequency4 ==
  PLL (3ph)1 : powerlib_meascontrol/PLL/PLL (3ph)  Commented=on  Fmin=45  Par_Init=[0, f]  ParK=[180, 3200, 1]  TcD=1e-4  MaxRateChangeFreq=12  FilterCutOffFreq=25  Ts=0  AGC=on
  "Power (3ph, Instantaneous)1" : powerlib_meascontrol/Measurements/Power (3ph, Instantaneous)
      settings: SourceProductName=Simscape Power Systems
  F (Hz) : Outport
  P (W) : Outport  Port=2
  wires:
  [I_ac_dfig_low] -> "Power (3ph, Instantaneous)1"/2
  PLL (3ph)1/1 -> F (Hz)/1
  "Power (3ph, Instantaneous)1"/1 -> P (W)/1  "Pot"
  [V_ac_dfig_low] -> PLL (3ph)1/1, "Power (3ph, Instantaneous)1"/1

== system DFIG_and_BESS_Voltae_Control/Measurement of Power - Frequency5 ==
  PLL (3ph)1 : powerlib_meascontrol/PLL/PLL (3ph)  Fmin=45  Par_Init=[0, f]  ParK=[180, 3200, 1]  TcD=1e-4  MaxRateChangeFreq=12  FilterCutOffFreq=25  Ts=0  AGC=on
  "Power (3ph, Instantaneous)1" : powerlib_meascontrol/Measurements/Power (3ph, Instantaneous)
      settings: SourceProductName=Simscape Power Systems
  F (Hz) : Outport
  P (W) : Outport  Port=2
  wires:
  [V_ac_syn_slack] -> "Power (3ph, Instantaneous)1"/1, PLL (3ph)1/1
  "Power (3ph, Instantaneous)1"/1 -> P (W)/1  "Pot"
  PLL (3ph)1/1 -> F (Hz)/1
  [I_ac_syn_slack] -> "Power (3ph, Instantaneous)1"/2

== system DFIG_and_BESS_Voltae_Control/Measurement of Power - Frequency6 ==
  PLL (3ph)1 : powerlib_meascontrol/PLL/PLL (3ph)  Commented=on  Fmin=45  Par_Init=[0, f]  ParK=[180, 3200, 1]  TcD=1e-4  MaxRateChangeFreq=12  FilterCutOffFreq=25  Ts=0  AGC=on
  "Power (3ph, Instantaneous)1" : powerlib_meascontrol/Measurements/Power (3ph, Instantaneous)
      settings: SourceProductName=Simscape Power Systems
  F (Hz) : Outport
  P (W) : Outport  Port=2
  wires:
  [V_ac_line_4] -> "Power (3ph, Instantaneous)1"/1, PLL (3ph)1/1
  "Power (3ph, Instantaneous)1"/1 -> P (W)/1  "Pot"
  PLL (3ph)1/1 -> F (Hz)/1
  [I_ac_line_4] -> "Power (3ph, Instantaneous)1"/2

== system DFIG_and_BESS_Voltae_Control/Measurement of Power - Frequency7 ==
  PLL (3ph)1 : powerlib_meascontrol/PLL/PLL (3ph)  Commented=on  Fmin=45  Par_Init=[0, f]  ParK=[180, 3200, 1]  TcD=1e-4  MaxRateChangeFreq=12  FilterCutOffFreq=25  Ts=0  AGC=on
  "Power (3ph, Instantaneous)1" : powerlib_meascontrol/Measurements/Power (3ph, Instantaneous)
      settings: SourceProductName=Simscape Power Systems
  F (Hz) : Outport
  P (W) : Outport  Port=2
  wires:
  [I_ac_load] -> "Power (3ph, Instantaneous)1"/2
  PLL (3ph)1/1 -> F (Hz)/1
  "Power (3ph, Instantaneous)1"/1 -> P (W)/1  "Pot"
  [V_ac_load] -> PLL (3ph)1/1, "Power (3ph, Instantaneous)1"/1

== system DFIG_and_BESS_Voltae_Control/Measurement of Power - Frequency8 ==
  PLL (3ph)1 : powerlib_meascontrol/PLL/PLL (3ph)  Commented=on  Fmin=45  Par_Init=[0, f]  ParK=[180, 3200, 1]  TcD=1e-4  MaxRateChangeFreq=12  FilterCutOffFreq=25  Ts=0  AGC=on
  "Power (3ph, Instantaneous)1" : powerlib_meascontrol/Measurements/Power (3ph, Instantaneous)
      settings: SourceProductName=Simscape Power Systems
  F (Hz) : Outport
  P (W) : Outport  Port=2
  wires:
  [I_ac_line_3] -> "Power (3ph, Instantaneous)1"/2
  PLL (3ph)1/1 -> F (Hz)/1
  "Power (3ph, Instantaneous)1"/1 -> P (W)/1  "Pot"
  [V_ac_line_3] -> PLL (3ph)1/1, "Power (3ph, Instantaneous)1"/1

== system DFIG_and_BESS_Voltae_Control/Measurement of Power - Frequency9 ==
  PLL (3ph)1 : powerlib_meascontrol/PLL/PLL (3ph)  Fmin=45  Par_Init=[0, f]  ParK=[180, 3200, 1]  TcD=1e-4  MaxRateChangeFreq=12  FilterCutOffFreq=25  Ts=0  AGC=on
  "Power (3ph, Instantaneous)1" : powerlib_meascontrol/Measurements/Power (3ph, Instantaneous)
      settings: SourceProductName=Simscape Power Systems
  F (Hz) : Outport
  P (W) : Outport  Port=2
  wires:
  [I_ac_bat_low] -> "Power (3ph, Instantaneous)1"/2
  PLL (3ph)1/1 -> F (Hz)/1
  "Power (3ph, Instantaneous)1"/1 -> P (W)/1  "Pot"
  [V_ac_bat_low] -> PLL (3ph)1/1, "Power (3ph, Instantaneous)1"/1

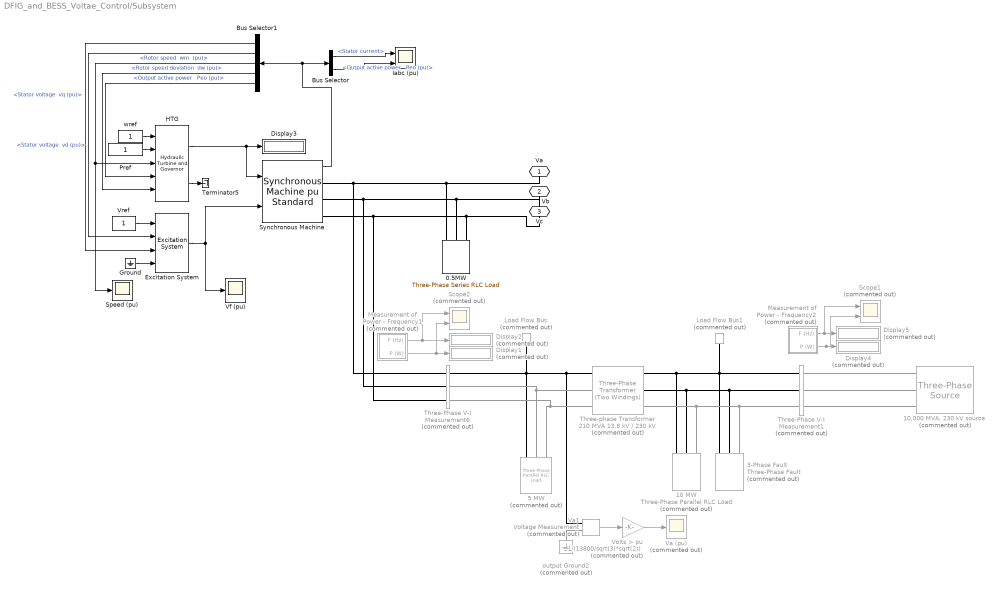
== system DFIG_and_BESS_Voltae_Control/Subsystem ==
  " Iabc (pu)" : Scope  NumInputPorts=2
  " Speed (pu)" : Scope
  0.5MW : powerlib/Elements/Three-Phase Series RLC Load  LConnTagsString=A|B|C  Configuration=Y (grounded)  NominalVoltage=13800  Vabc=[1e3 1e3 1e3]  Vabcp=[1e3 1e3 1e3]  NominalFrequency=f  UnbalancedPower=off  ActivePower=0.5e6  InductivePower=0  CapacitivePower=0  Pabc=[10e3 9e3 11e3]  QLabc=[100 90 110]  QCabc=[100 90 110]  Pabcp=[10e3 9e3 11e3]  QLabcp=[100 90 110]  QCabcp=[100 90 110]  Measurements=None  LoadType=constant Z
  10 MW : powerlib/Elements/Three-Phase Parallel RLC Load  Commented=on  LConnTagsString=A|B|C  Configuration=Y (grounded)  NominalVoltage=230e3  Vabc=[1e3 1e3 1e3]  Vabcp=[1e3 1e3 1e3]  NominalFrequency=f  UnbalancedPower=off  ActivePower=10000000  InductivePower=0  CapacitivePower=0  Pabc=[10e3 9e3 11e3]  QLabc=[100 90 110]  QCabc=[100 90 110]  Pabcp=[10e3 9e3 11e3]  QLabcp=[100 90 110]  QCabcp=[100 90 110]  Measurements=None  LoadType=constant Z
  "10,000 MVA, 230 kV source" : powerlib/Electrical Sources/Three-Phase Source  Commented=on  InternalConnection=Yg  VoltagePhases=off  Voltage=(230000)*1.00006  PhaseAngle=-0.77547  Voltage_phases=[25e3 25e3 25e3]/sqrt(3)  PhaseAngles_phases=[0 -120 +120]  Frequency=60  NonIdealSource=on  SpecifyImpedance=on  Resistance=0.529  Inductance=0.0140  ShortCircuitLevel=10000e6  BaseVoltage=230e3  XRratio=10  BusType=swing  Pref=0  Qref=0  Prefabc=[10e3, 10e3, 10e3]  Qrefabc=[0, 0, 0]  Qmin=-Inf  Qmax=Inf
  3-Phase Fault : powerlib/Elements/Three-Phase Fault  Commented=on  InitialStates=0  FaultA=on  FaultB=on  FaultC=on  GroundFault=on  SwitchTimes=[ 0.1 0.2]  External=off  SwitchStatus=NaN  FaultResistance=1e-3  GroundResistance=1e-3  SnubberResistance=inf  SnubberCapacitance=inf  Measurements=None
  5 MW : powerlib/Elements/Three-Phase Parallel RLC Load  Commented=on  LConnTagsString=A|B|C  Configuration=Y (grounded)  NominalVoltage=13.8e3  Vabc=[1e3 1e3 1e3]  Vabcp=[1e3 1e3 1e3]  NominalFrequency=60  UnbalancedPower=off  ActivePower=5000000  InductivePower=0  CapacitivePower=0  Pabc=[10e3 9e3 11e3]  QLabc=[100 90 110]  QCabc=[100 90 110]  Pabcp=[10e3 9e3 11e3]  QLabcp=[100 90 110]  QCabcp=[100 90 110]  Measurements=None  LoadType=constant Z
  Bus Selector : BusSelector  OutputSignals="Stator current,Output active power   Peo (pu)"
  Bus Selector1 : BusSelector  OutputSignals="dq0 components.Stator voltage  vq (pu),dq0 components.Stator voltage  vd (pu),Mechanical.Rotor speed  wm  (pu),Mechanical.Rotor speed deviation  dw (pu),Output active power   Peo (pu)"
  Display{1..2,4..5} (4 alike) : Display  Commented=on
  Display3 : Display
  Excitation System : sps_avr/Excitation System  tr=20e-3  reg=[ 300, 0.001 ]  exc=[ 1, 0 ]  tgr=[ 0, 0 ]  damp=[ 0.001, 0.1 ]  sat=[ 0, 0 ]  lim=[ -11.5, 11.5, 0 ]  v0=[1,1.29071]
      settings: SourceProductName=Simscape Power Systems  SourceProductBaseCode=PS
  Ground : Ground
  HTG : powerlib/Machines/Hydraulic Turbine and Governor  sm="[ 10/3  0.07 ]"  gate="[  0.01  0.97518  -0.1  0.1 ]"  reg="[  0.05  1.163  0.105  0  0.01  ]"  hyd="[  0  2.67  ]"  dref=0  po=1
      settings: SourceProductName=Simscape Power Systems  SourceProductBaseCode=PS
  Load Flow Bus : powerlib/Measurements/Load Flow Bus  Commented=on  LConnTagsString=a  Phases=single  Connectors=on one side  ID=B1  Vbase=13.8e3  Vref=1  Vangle=0  VLF=1  VLFb=1  VLFc=1  angleLF=-23.67  angleLFb=0  angleLFc=0
      settings: AttributesFormatString=%<ID>\n%<Vbase>V\n%<VLF>pu\n%<angleLF>deg.  SourceProductName=Simscape Power Systems
  Load Flow Bus1 : powerlib/Measurements/Load Flow Bus  Commented=on  LConnTagsString=a  Phases=single  Connectors=on one side  ID=B2  Vbase=230e3  Vref=1  Vangle=0  VLF=1  VLFb=1  VLFc=1  angleLF=0  angleLFb=0  angleLFc=0
      settings: AttributesFormatString=%<ID>\n%<Vbase>V\n%<VLF>pu\n%<angleLF>deg.  SourceProductName=Simscape Power Systems
  Measurement of Power - Frequency1 : Subsystem  Commented=on
  Measurement of Power - Frequency2 : Subsystem  Commented=on
  Pref : Constant
  Scope1 : Scope  Commented=on  NumInputPorts=2
  Scope2 : Scope  Commented=on  NumInputPorts=2
  "Synchronous Machine " : powerlib/Machines/Synchronous Machine pu Standard  PresetModel=No  MechanicalLoad=Mechanical power Pm  ShowDetailedParameters=on  RotorType=Salient-pole  Units=per unit standard parameters  MeasurementBus=off  NominalParameters="[ 7.5e6  13800   f ]"  Reactances1=[ 31 32 33 34 35 36 37 ]  Reactances2=[ 1.305, 0.296, 0.252, 0.474, 0.243, 0.18 ]  dAxisTimeConstants=Short-circuit  qAxisTimeConstants=Open-circuit  TimeConstants1=[]  TimeConstants2=[]  TimeConstants3=[]  TimeConstants4=[]  TimeConstants5=[ 1.01, 0.053, 0.1 ]  TimeConstants6=[]  TimeConstants7=[]  TimeConstants8=[]  StatorResistance=2.8544e-3  Mechanical=[ 3.2 0 2]  PolePairs=2  InitialConditions=[0 -94.2826 0.750185 0.750185 0.750185 -24.943 -144.943 95.057 1.29071]  SetSaturation=off  Saturation=[0.6404,0.7127,0.8441,0.9214,0.9956,1.082,1.19,1.316,1.457;0.7,0.7698,0.8872,0.9466,0.9969,1.046,1.1,1.151,1.201]  LoadFlowParameters=[1 150000000 0 0]  TsPowergui=0  TsBlock=-1  IterativeModel=Trapezoidal non iterative  IterativeDiscreteModel=Trapezoidal non iterative  BusType=PV  Pref=150000000  Qref=0  Qmin=-Inf  Qmax=Inf  PLF=0  QLF=0
      settings: AttributesFormatString=\n\n  SourceProductName=Simscape Power Systems
  Terminator5 : Terminator
  Three-Phase V-I Measurement1 : powerlib/Measurements/Three-Phase V-I Measurement  Commented=on  VoltageMeasurement=phase-to-ground  SetLabelV=on  LabelV=V_ac_syn_low2  Vpu=off  VpuLL=off  CurrentMeasurement=yes  SetLabelI=on  LabelI=I_ac_syn_low2  Ipu=off  Pbase=100e6  Vbase=500e3  OutputType=Complex  PhasorSimulation=off  PSBequivalent=0
  Three-Phase V-I Measurement6 : powerlib/Measurements/Three-Phase V-I Measurement  Commented=on  VoltageMeasurement=phase-to-ground  SetLabelV=on  LabelV=V_ac_syn_low1  Vpu=off  VpuLL=off  CurrentMeasurement=yes  SetLabelI=on  LabelI=I_ac_syn_low1  Ipu=off  Pbase=100e6  Vbase=500e3  OutputType=Complex  PhasorSimulation=off  PSBequivalent=0
  Three-phase Transformer 210 MVA 13.8 kV / 230 kV : powerlib/Elements/Three-Phase Transformer (Two Windings)  Commented=on  Winding1Connection=Delta (D1)  Winding2Connection=Yg  CoreType=Three single-phase transformers  SetSaturation=off  Hysteresis=off  DataFile='hysteresis'  SetInitialFlux=off  Measurements=None  UNITS=pu  NominalPower=[ 210e6 60 ]  Winding1="[ 13.8e3 0.0027  0.08]"  Winding2=[ 230e3 0.0027 0.08]  Rm=500  Lm=500  L0=0.5  Saturation="[ 0,0  ;  0.005,1.2  ;  1.0,1.4 ]"  InitialFluxes=[ 0.8 , -0.8 , 0.7 ]  MoreParameters=off  BreakLoop=off  DataType=off  TransfoNumber=0
  Va (pu) : Scope  Commented=on
  Va1 : powerlib/Measurements/Voltage Measurement  Tag=PoWeRsYsTeMmEaSuReMeNt  Commented=on  PhasorSimulation=off  OutputType=Magnitude  PSBequivalent=0
  Vf (pu) : Scope
  Volts > pu : Gain  Commented=on  Gain=1/(13800/sqrt(3)*sqrt(2))  SaturateOnIntegerOverflow=on  OutDataTypeStr=Inherit: Same as input  ParamDataTypeStr=Inherit: Same as input
  Vref : Constant
  output Ground2 : powerlib/Elements/Ground  Commented=on  LConnTagsString=a
  wref : Constant
  Va : PMIOPort  Port=1  Side=Left
  Vb : PMIOPort  Port=2  Side=Left
  Vc : PMIOPort  Port=3  Side=Left
  wires:
  Bus Selector1/5 -> HTG/4  "<Output active power   Peo (pu)>"
  HTG/2 -> Terminator5/1
  Bus Selector1/3 -> HTG/3, " Speed (pu)"/1  "<Rotor speed  wm  (pu)>"
  Bus Selector/1 -> " Iabc (pu)"/1  "<Stator current>"
  Bus Selector1/2 -> Excitation System/2  "<Stator voltage  vd (pu)>"
  Ground/1 -> Excitation System/4
  Bus Selector1/1 -> Excitation System/3  "<Stator voltage  vq (pu)>"
  Va1/1 -> Volts > pu/1
  Excitation System/1 -> Vf (pu)/1, "Synchronous Machine "/2
  Bus Selector1/4 -> HTG/5  "<Rotor speed deviation  dw (pu)>"
  Volts > pu/1 -> Va (pu)/1
  Pref/1 -> HTG/2
  wref/1 -> HTG/1
  Vref/1 -> Excitation System/1
  "Synchronous Machine "/1 -> Bus Selector/1, Bus Selector1/1
  Measurement of Power - Frequency1/1(F (Hz)) -> Scope2/1, Display2/1
  Measurement of Power - Frequency1/2(P (W)) -> Scope2/2, Display1/1
  Bus Selector/2 -> " Iabc (pu)"/2  "<Output active power   Peo (pu)>"
  HTG/1 -> "Synchronous Machine "/1, Display3/1
  Measurement of Power - Frequency2/1(F (Hz)) -> Scope1/1, Display5/1
  Measurement of Power - Frequency2/2(P (W)) -> Scope1/2, Display4/1
  connections:
  Va1/LConn1 -- Three-Phase V-I Measurement6/RConn1 -- 5 MW/LConn1 -- Load Flow Bus/LConn1 -- Three-phase Transformer 210 MVA 13.8 kV / 230 kV/LConn1
  5 MW/LConn3 -- Three-Phase V-I Measurement6/RConn3 -- Three-phase Transformer 210 MVA 13.8 kV / 230 kV/LConn3
  10 MW/LConn2 -- Three-phase Transformer 210 MVA 13.8 kV / 230 kV/RConn2 -- Three-Phase V-I Measurement1/LConn2 -- 3-Phase Fault/LConn2
  Load Flow Bus1/LConn1 -- Three-phase Transformer 210 MVA 13.8 kV / 230 kV/RConn1 -- 10 MW/LConn1 -- Three-Phase V-I Measurement1/LConn1 -- 3-Phase Fault/LConn1
  3-Phase Fault/LConn3 -- Three-Phase V-I Measurement1/LConn3 -- Three-phase Transformer 210 MVA 13.8 kV / 230 kV/RConn3 -- 10 MW/LConn3
  5 MW/LConn2 -- Three-Phase V-I Measurement6/RConn2 -- Three-phase Transformer 210 MVA 13.8 kV / 230 kV/LConn2
  output Ground2/LConn1 -- Va1/LConn2
  0.5MW/LConn1 -- Three-Phase V-I Measurement6/LConn1 -- "Synchronous Machine "/RConn1 -- Va/RConn1
  Vb/RConn1 -- "Synchronous Machine "/RConn2 -- Three-Phase V-I Measurement6/LConn2 -- 0.5MW/LConn2
  0.5MW/LConn3 -- "Synchronous Machine "/RConn3 -- Three-Phase V-I Measurement6/LConn3 -- Vc/RConn1
  Three-Phase V-I Measurement1/RConn1 -- "10,000 MVA, 230 kV source"/RConn1
  Three-Phase V-I Measurement1/RConn2 -- "10,000 MVA, 230 kV source"/RConn2
  Three-Phase V-I Measurement1/RConn3 -- "10,000 MVA, 230 kV source"/RConn3
